simulink model "EV3_test_RST"  (Simulink 7.6)
settings: Solver=FixedStepDiscrete  StartTime=0.0  StopTime=Inf  RelTol=1e-3
libraries: rpi_blkst x1
settings Model: Creator=jacques  LastModifiedBy=jacques  SimulationMode=external
settings OptimizationCC: OptimizeModelRefInitCode=on  LifeSpan=1
settings HardwareCC: ProdLargestAtomicInteger=Long  ProdLargestAtomicFloat=Double  ProdEndianess=LittleEndian  ProdHWDeviceType=ARM Compatible->ARM 11
settings RTWCC: SystemTargetFile=ert_rpi.tlc  TemplateMakefile=ert_rpi.tmf  PostCodeGenCommand=postGenFunc(buildInfo)  Description=RTW Embedded Coder RPI target  ProcessScript=ert_rpi_make_rtw_hook
settings CodeAppCC: IgnoreCustomStorageClasses=off
settings STFCustomTargetCC: ModelReferenceCompliant=off  CombineOutputUpdateFcns=on  ERTCustomFileBanners=on  SupportNonInlinedSFcns=off  SystemTargetFile=ert_rpi.tlc
settings ERTTargetCC: MultiwordLength=2048  ModelReferenceCompliant=off  ParMdlRefBuildCompliant=off  CompOptLevelCompliant=off  ERTFirstTimeCompliant=off  SupportContinuousTime=on  ModelStepFunctionPrototypeControlCompliant=off  CPPClassGenCompliant=off  ExtMode=on  ExtModeMexArgs='192.168.2.1'  InlinedParameterPlacement=NonHierarchical  ERTCustomFileTemplate=ert_rpi_file_process.tlc  ConvertIfToSwitch=off

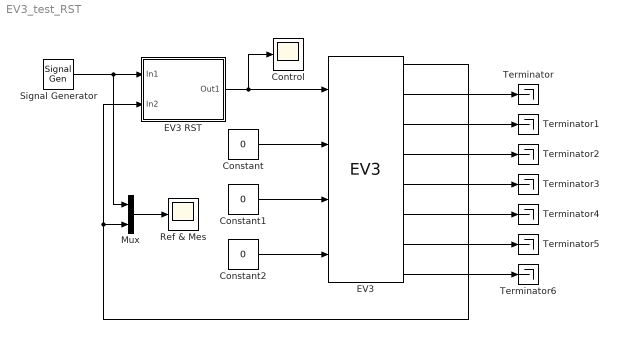
== system EV3_test_RST ==
  Constant : Constant  Value=0  SampleTime=0.01
  Constant1 : Constant  Value=0  SampleTime=0.01
  Constant2 : Constant  Value=0  SampleTime=0.01
  Control : Scope
      settings: YMin=-12.5  YMax=15
  EV3 : rpi_blkst/EV3  SystemSampleTime=-1  rpi_mask_Ts=0.01
  EV3 RST : Subsystem
      mask Type: EV3 RST
      mask Description: RST position controller for EV3 motors
      mask Help:
      | This RST controller is tuned to follow accurately class 2 references.
      | Its sampling period is fixed and equal to 0.01s.
      | It is suited for the big motors: NXT motors and EV3 big motors.
      mask Display:
      | disp('RST')
      | port_label('input',1,'Ref')
      | port_label('input',2,'Mes')
      | port_label('output',1,'U')
  Mux : Mux  Inputs=2
  Ref & Mes : Scope
      settings: YMin=-45  YMax=45
  Signal Generator : SignalGenerator  Amplitude=0  Frequency=0.5
  Terminator{,1..6} (7 alike) : Terminator
  wires:
  EV3 RST/1(Out1) -> EV3/1, Control/1
  EV3/1 -> EV3 RST/2(In2), Mux/2
  EV3/2 -> Terminator/1
  EV3/3 -> Terminator1/1
  EV3/4 -> Terminator2/1
  EV3/5 -> Terminator3/1
  EV3/6 -> Terminator4/1
  EV3/7 -> Terminator5/1
  EV3/8 -> Terminator6/1
  Constant/1 -> EV3/2
  Constant1/1 -> EV3/3
  Constant2/1 -> EV3/4
  Signal Generator/1 -> EV3 RST/1(In1), Mux/1
  Mux/1 -> Ref & Mes/1

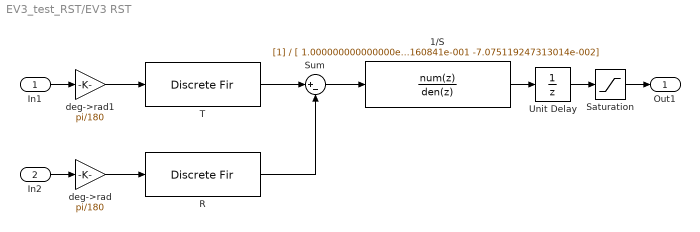
== system EV3_test_RST/EV3 RST ==
  In1 : Inport
  In2 : Inport  Port=2
  1/S : DiscreteFilter  Denominator=[ 1.000000000000000e+000 -1.397430293642954e+000 4.681814861160841e-001 -7.075119247313014e-002]  SampleTime=0.01  a0EqualsOne=on
  R : DiscreteFir  NumCoeffs=[6.915174485840503e+002 -1.259172933566519e+003 5.714958970624333e+002]  SampleTime=0.01
  Saturation : Saturate  UpperLimit=100  LowerLimit=-100  SampleTime=0.01
  Sum : Sum  Inputs=|+-
  T : DiscreteFir  NumCoeffs=[1.181478528937075e+004 -4.112324830972540e+004 5.385298179536037e+004 -3.146381703126604e+004 6.923138668340286e+003]  SampleTime=0.01
  Unit Delay : UnitDelay  SampleTime=0.01
  deg->rad : Gain  Gain=pi/180  SampleTime=0.01
  deg->rad1 : Gain  Gain=pi/180  SampleTime=0.01
  Out1 : Outport
  wires:
  T/1 -> Sum/1
  Sum/1 -> 1/S/1
  1/S/1 -> Unit Delay/1
  Unit Delay/1 -> Saturation/1
  R/1 -> Sum/2
  Saturation/1 -> Out1/1
  In1/1 -> deg->rad1/1
  In2/1 -> deg->rad/1
  deg->rad/1 -> R/1
  deg->rad1/1 -> T/1
